simulink model "ex_model_B"  (R2022b)
settings: Solver=FixedStepAuto  StartTime=0.0  StopTime=10.0  RelTol=1e-3
undefined symbols (not defined in the file): T1Break, T1Data, T2Break, T2Data
settings Model: Creator=amyyang  LastModifiedBy=amyyang
settings OptimizationCC: DefaultParameterBehavior=Inlined  EnhancedBackFolding=on  PassReuseOutputArgsAs=Individual arguments  ZeroExternalMemoryAtStartup=off  ZeroInternalMemoryAtStartup=off  OptimizeBlockOrder=speed  DifferentSizesBufferReuse=on  OptimizationCustomize=off  EfficientTunableParamExpr=on
settings DebuggingCC: ParameterTunabilityLossMsg=error
settings ModelReferenceCC: ModelReferenceNumInstancesAllowed=Single
settings SFSimCC: MATLABDynamicMemAlloc=off
settings RTWCC: Description=Embedded Coder  SystemTargetFile=ert.tlc  TemplateMakefile=ert_default_tmf  Toolchain=LCC-win64 v2.4.1 | gmake (64-bit Windows)
settings CodeAppCC: ForceParamTrailComments=on  IgnoreCustomStorageClasses=off  MaxIdLength=256  OperatorAnnotations=on  SimulinkDataObjDesc=on  SFDataObjDesc=on  InsertBlockDesc=on
settings ERTTargetCC: TargetLangStandard=C99 (ISO)  GenerateSampleERTMain=on  InlinedParameterPlacement=NonHierarchical  ERTCustomFileTemplate=example_file_process.tlc

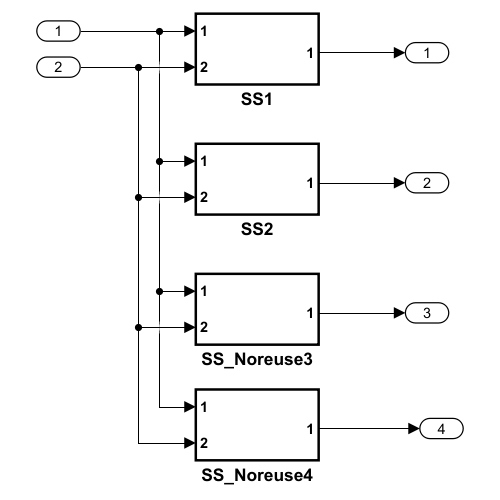
[thumbnail: Simulink's stored preview of the top-level diagram]
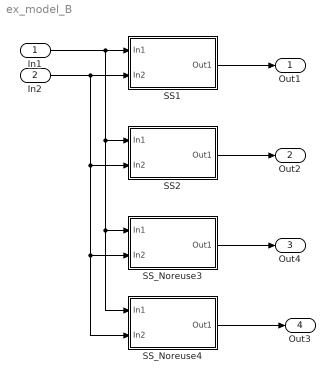
== system ex_model_B ==
  In1 : Inport
  In2 : Inport  Port=2
  SS1 : Subsystem  TreatAsAtomicUnit=on  RTWFcnName=myfun  RTWFileName=myfile  mask(SSDemo){x=T1Break, y=T1Data}
      mask prompts: x "Break points (X data):"; y "Output values (Y data):"
      mask help: Example to show code reuse. This example has two parameters for a lookup table.
  SS2 : Subsystem  TreatAsAtomicUnit=on  RTWFcnName=myfun  RTWFileName=myfile  mask(SSDemo){x=T2Break, y=T2Data}
      mask prompts: x "Break points (X data):"; y "Output values (Y data):"
      mask help: Example to show code reuse. This example has two parameters for a lookup table.
  SS_Noreuse3 : Subsystem  TreatAsAtomicUnit=on  RTWFcnName=myfun_Fixed  RTWFileName=myfileFixed  mask(SSDemo){x=T2Break, y=T2Data}
      mask prompts: x "Break points (X data):"; y "Output values (Y data):"
      mask help: Example to show code reuse. This example has two parameters for a lookup table.
      settings: RTWSystemCode=Nonreusable function  FunctionInterfaceSpec=Allow arguments (Match graphical interface)
  SS_Noreuse4 : Subsystem  TreatAsAtomicUnit=on  RTWFcnName=myfun_Fixed  RTWFileName=myfileFixed  mask(SSDemo){x=T2Break, y=T2Data}
      mask prompts: x "Break points (X data):"; y "Output values (Y data):"
      mask help: Example to show code reuse. This example has two parameters for a lookup table.
      settings: RTWSystemCode=Nonreusable function  FunctionInterfaceSpec=Allow arguments (Match graphical interface)
  Out1 : Outport
  Out2 : Outport  Port=2
  Out4 : Outport  Port=3
  Out3 : Outport  Port=4
  wires:
  In1/1 -> SS2/1(In1), SS_Noreuse4/1(In1), SS_Noreuse3/1(In1), SS1/1(In1)
  In2/1 -> SS_Noreuse4/2(In2), SS_Noreuse3/2(In2), SS2/2(In2), SS1/2(In2)
  SS1/1(Out1) -> Out1/1
  SS2/1(Out1) -> Out2/1
  SS_Noreuse3/1(Out1) -> Out4/1
  SS_Noreuse4/1(Out1) -> Out3/1

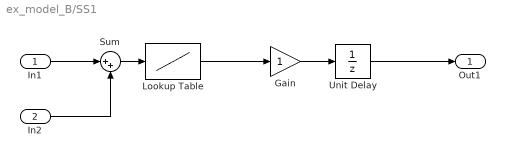
== system ex_model_B/SS1 ==
  In1 : Inport  OutDataTypeStr=double
  In2 : Inport  Port=2  OutDataTypeStr=double
  Gain : Gain
  Lookup Table : Lookup_n-D  NumberOfTableDimensions=1  BreakpointsForDimension1=x  Table=y
  Sum : Sum  Inputs=|++
  Unit Delay : UnitDelay  SampleTime=-1  HasFrameUpgradeWarning=on
  Out1 : Outport  OutDataTypeStr=double  VectorParamsAs1DForOutWhenUnconnected=off
  wires:
  Gain/1 -> Unit Delay/1
  Lookup Table/1 -> Gain/1
  In1/1 -> Sum/1
  In2/1 -> Sum/2
  Sum/1 -> Lookup Table/1
  Unit Delay/1 -> Out1/1

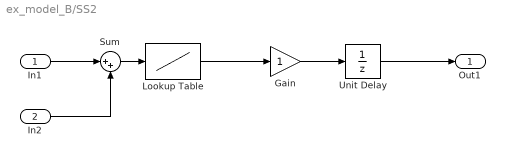
== system ex_model_B/SS2 ==
  In1 : Inport  OutDataTypeStr=double
  In2 : Inport  Port=2  OutDataTypeStr=double
  Gain : Gain
  Lookup Table : Lookup_n-D  NumberOfTableDimensions=1  BreakpointsForDimension1=x  Table=y
  Sum : Sum  Inputs=|++
  Unit Delay : UnitDelay  SampleTime=-1  HasFrameUpgradeWarning=on
  Out1 : Outport  OutDataTypeStr=double  VectorParamsAs1DForOutWhenUnconnected=off
  wires:
  Sum/1 -> Lookup Table/1
  In2/1 -> Sum/2
  In1/1 -> Sum/1
  Lookup Table/1 -> Gain/1
  Gain/1 -> Unit Delay/1
  Unit Delay/1 -> Out1/1

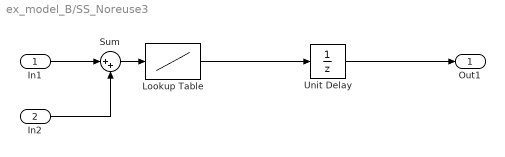
== system ex_model_B/SS_Noreuse3 ==
  In1 : Inport
  In2 : Inport  Port=2
  Lookup Table : Lookup_n-D  NumberOfTableDimensions=1  BreakpointsForDimension1=x  Table=y
  Sum : Sum  Inputs=|++
  Unit Delay : UnitDelay  SampleTime=-1  HasFrameUpgradeWarning=on
  Out1 : Outport  VectorParamsAs1DForOutWhenUnconnected=off
  wires:
  Sum/1 -> Lookup Table/1
  In2/1 -> Sum/2
  In1/1 -> Sum/1
  Lookup Table/1 -> Unit Delay/1
  Unit Delay/1 -> Out1/1

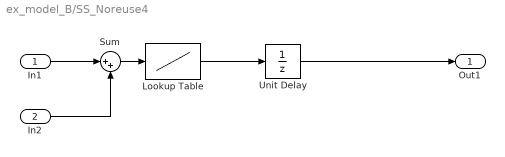
== system ex_model_B/SS_Noreuse4 ==
  In1 : Inport
  In2 : Inport  Port=2
  Lookup Table : Lookup_n-D  NumberOfTableDimensions=1  BreakpointsForDimension1=x  Table=y
  Sum : Sum  Inputs=|++
  Unit Delay : UnitDelay  SampleTime=-1  HasFrameUpgradeWarning=on
  Out1 : Outport  VectorParamsAs1DForOutWhenUnconnected=off
  wires:
  Lookup Table/1 -> Unit Delay/1
  In1/1 -> Sum/1
  In2/1 -> Sum/2
  Sum/1 -> Lookup Table/1
  Unit Delay/1 -> Out1/1
